simulink subsystem "EM"  (R2024a)
settings: Solver=VariableStepAuto  StartTime=0.0  StopTime=10.0  RelTol=1e-3
settings Model: Creator=Dell  LastModifiedBy=mrvol

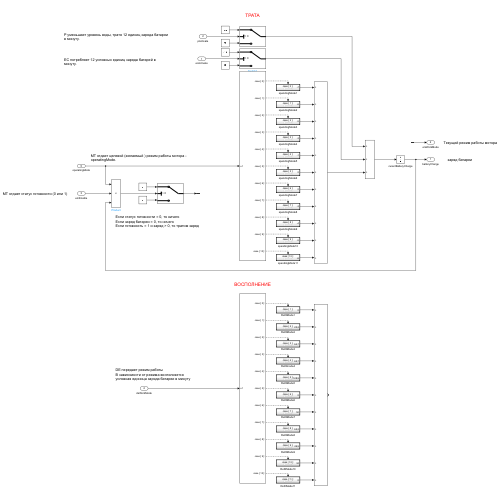
[thumbnail: Simulink's stored preview of the top-level diagram]
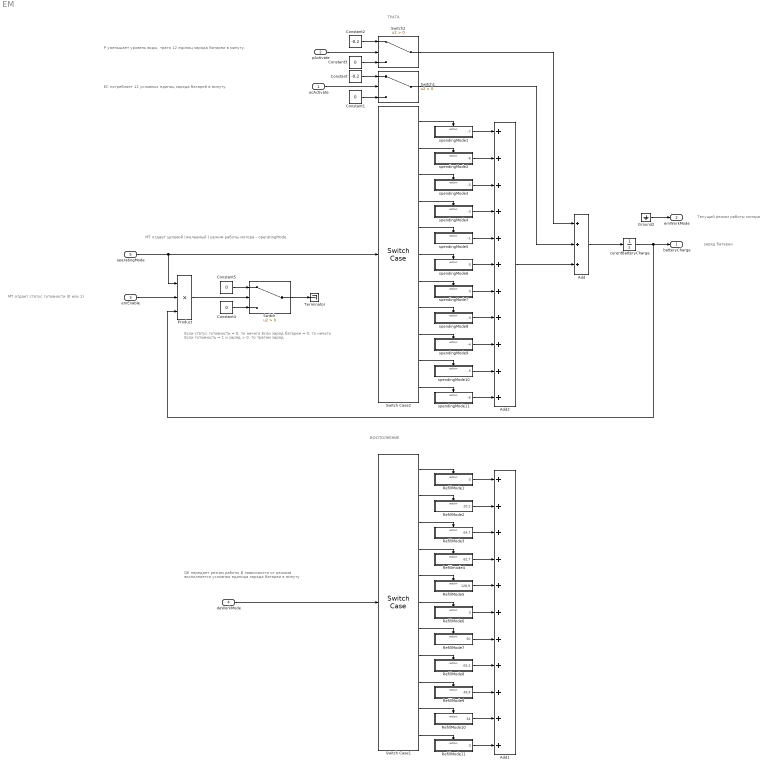
== system EM ==
  note: Если статус готовности = 0, то ничего
      | Если заряд батареи = 0, то ничего
      | Если готовность = 1 и заряд > 0, то тратим заряд
  note: ВОСПОЛНЕНИЕ
  note: ТРАТА
  note: EC потребляет 12 условных единиц заряда батарей в минуту.
  note: Текущий режим работы мотора
  note: заряд батареи
  note: P уменьшает уровень воды, тратя 12 единиц заряда батареи в минуту.
  note: MT отдает статус готовности (0 или 1)
  note: MT отдает целевой (желаемый ) режим работы мотора - operatingMode.
  note: DE передает режим работы
      | В зависомости от режима восполняется
      | условная единица заряда батареи в минуту
  ecActivate : Inport
  pActivate : Inport  Port=2
  emEnable : Inport  Port=3
  deWorkMode : Inport  Port=4
  operatingMode : Inport  Port=5
  Add : Sum  Inputs=+++
  Add1 : Sum  Inputs=+++++++++++
  Add2 : Sum  Inputs=+++++++++++
  Constant : Constant  Value=-0.2
  Constant{1,3..5} (4 alike) : Constant  Value=0
  Constant2 : Constant  Value=-0.2
  Ground2 : Ground
  Product : Product  Inputs=3
  RefillMode1 : Subsystem  TreatAsAtomicUnit=on
  RefillMode10 : Subsystem  TreatAsAtomicUnit=on
  RefillMode11 : Subsystem  TreatAsAtomicUnit=on
  RefillMode2 : Subsystem  TreatAsAtomicUnit=on
  RefillMode3 : Subsystem  TreatAsAtomicUnit=on
  RefillMode5 : Subsystem  TreatAsAtomicUnit=on
  RefillMode6 : Subsystem  TreatAsAtomicUnit=on
  RefillMode7 : Subsystem  TreatAsAtomicUnit=on
  RefillMode8 : Subsystem  TreatAsAtomicUnit=on
  RefillMode9 : Subsystem  TreatAsAtomicUnit=on
  Refillmode4 : Subsystem  TreatAsAtomicUnit=on
  Switch : Switch  Criteria=u2 > Threshold  SaturateOnIntegerOverflow=off  InputSameDT=off
  Switch Case1 : SwitchCase  CaseConditions={0, 1, 2, 3, 4, 5, 6, 7, 8, 9, 10}  ShowDefaultCase=off
  Switch Case2 : SwitchCase  CaseConditions={0, 1, 2, 3, 4, 5, 6, 7, 8, 9, 10}  ShowDefaultCase=off
  Switch1 : Switch  Criteria=u2 > Threshold  SaturateOnIntegerOverflow=off  InputSameDT=off
  Switch2 : Switch  Criteria=u2 > Threshold  SaturateOnIntegerOverflow=off  InputSameDT=off
  Terminator : Terminator
  curentBatteryCharge : Integrator
  spendingMode1 : Subsystem  TreatAsAtomicUnit=on
  spendingMode10 : Subsystem  TreatAsAtomicUnit=on
  spendingMode11 : Subsystem  TreatAsAtomicUnit=on
  spendingMode2 : Subsystem  TreatAsAtomicUnit=on
  spendingMode3 : Subsystem  TreatAsAtomicUnit=on
  spendingMode4 : Subsystem  TreatAsAtomicUnit=on
  spendingMode5 : Subsystem  TreatAsAtomicUnit=on
  spendingMode6 : Subsystem  TreatAsAtomicUnit=on
  spendingMode7 : Subsystem  TreatAsAtomicUnit=on
  spendingMode8 : Subsystem  TreatAsAtomicUnit=on
  spendingMode9 : Subsystem  TreatAsAtomicUnit=on
  batteryCharge : Outport
  emWorkMode : Outport  Port=2
  wires:
  Ground2/1 -> emWorkMode/1
  ecActivate/1 -> Switch1/2
  Constant/1 -> Switch1/1
  Constant1/1 -> Switch1/3
  pActivate/1 -> Switch2/2
  Constant2/1 -> Switch2/1
  Constant3/1 -> Switch2/3
  Constant4/1 -> Switch/3
  Constant5/1 -> Switch/1
  Refillmode4/1(62,7) -> Add1/4
  RefillMode8/1(65,2) -> Add1/8
  RefillMode5/1(128,9) -> Add1/5
  RefillMode2/1(20,2) -> Add1/2
  RefillMode3/1(64,7) -> Add1/3
  RefillMode6/1(0) -> Add1/6
  RefillMode10/1(34) -> Add1/10
  RefillMode9/1(49,9) -> Add1/9
  RefillMode1/1(0) -> Add1/1
  RefillMode7/1(50) -> Add1/7
  Switch Case1/7 -> RefillMode7/Action
  Switch Case1/5 -> RefillMode5/Action
  RefillMode11/1(0) -> Add1/11
  Switch Case1/3 -> RefillMode3/Action
  Switch Case1/11 -> RefillMode11/Action
  Switch Case1/8 -> RefillMode8/Action
  Switch Case1/6 -> RefillMode6/Action
  Switch Case1/4 -> Refillmode4/Action
  Switch Case1/1 -> RefillMode1/Action
  Switch Case1/10 -> RefillMode10/Action
  Switch Case1/9 -> RefillMode9/Action
  Switch Case1/2 -> RefillMode2/Action
  deWorkMode/1 -> Switch Case1/1
  Product/1 -> Switch/2
  Switch2/1 -> Add/1
  Switch1/1 -> Add/2
  Add/1 -> curentBatteryCharge/1
  Switch Case2/1 -> spendingMode1/Action
  Switch Case2/10 -> spendingMode10/Action
  Switch Case2/9 -> spendingMode9/Action
  spendingMode7/1(0) -> Add2/7
  Switch Case2/8 -> spendingMode8/Action
  Switch Case2/7 -> spendingMode7/Action
  Switch Case2/6 -> spendingMode6/Action
  Switch Case2/5 -> spendingMode5/Action
  Switch Case2/11 -> spendingMode11/Action
  Switch Case2/3 -> spendingMode3/Action
  Switch Case2/4 -> spendingMode4/Action
  spendingMode11/1(-6) -> Add2/11
  spendingMode9/1(-4) -> Add2/9
  spendingMode2/1(-6) -> Add2/2
  spendingMode1/1(-7) -> Add2/1
  spendingMode10/1(-5) -> Add2/10
  spendingMode6/1(0) -> Add2/6
  spendingMode3/1(-5) -> Add2/3
  spendingMode8/1(-3) -> Add2/8
  spendingMode4/1(-3) -> Add2/4
  Switch Case2/2 -> spendingMode2/Action
  spendingMode5/1(-1) -> Add2/5
  Add2/1 -> Add/3
  curentBatteryCharge/1 -> Product/3, batteryCharge/1
  operatingMode/1 -> Switch Case2/1, Product/1
  emEnable/1 -> Product/2
  Switch/1 -> Terminator/1

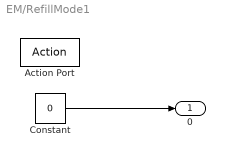
== system EM/RefillMode1 ==
  Action Port : ActionPort  ActionPortLabel=case [ 1 ]:
  Constant : Constant  Value=0
  0 : Outport
  wires:
  Constant/1 -> 0/1

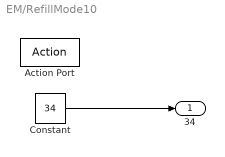
== system EM/RefillMode10 ==
  Action Port : ActionPort  ActionPortLabel=case [ 10 ]:
  Constant : Constant  Value=34
  34 : Outport
  wires:
  Constant/1 -> 34/1

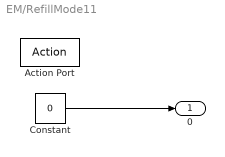
== system EM/RefillMode11 ==
  Action Port : ActionPort  ActionPortLabel=case [ 11 ]:
  Constant : Constant  Value=0
  0 : Outport
  wires:
  Constant/1 -> 0/1

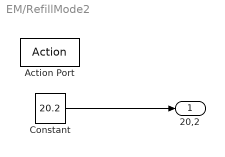
== system EM/RefillMode2 ==
  Action Port : ActionPort  ActionPortLabel=case [ 2 ]:
  Constant : Constant  Value=20.2
  20,2 : Outport
  wires:
  Constant/1 -> 20,2/1

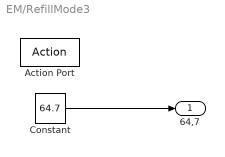
== system EM/RefillMode3 ==
  Action Port : ActionPort  ActionPortLabel=case [ 3 ]:
  Constant : Constant  Value=64.7
  64,7 : Outport
  wires:
  Constant/1 -> 64,7/1

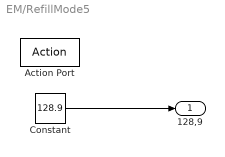
== system EM/RefillMode5 ==
  Action Port : ActionPort  ActionPortLabel=case [ 5 ]:
  Constant : Constant  Value=128.9
  128,9 : Outport
  wires:
  Constant/1 -> 128,9/1

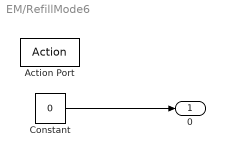
== system EM/RefillMode6 ==
  Action Port : ActionPort  ActionPortLabel=case [ 6 ]:
  Constant : Constant  Value=0
  0 : Outport
  wires:
  Constant/1 -> 0/1

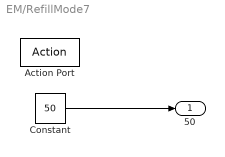
== system EM/RefillMode7 ==
  Action Port : ActionPort  ActionPortLabel=case [ 7 ]:
  Constant : Constant  Value=50
  50 : Outport
  wires:
  Constant/1 -> 50/1

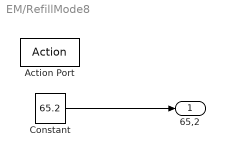
== system EM/RefillMode8 ==
  Action Port : ActionPort  ActionPortLabel=case [ 8 ]:
  Constant : Constant  Value=65.2
  65,2 : Outport
  wires:
  Constant/1 -> 65,2/1

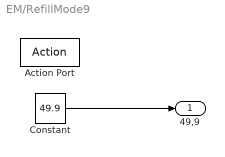
== system EM/RefillMode9 ==
  Action Port : ActionPort  ActionPortLabel=case [ 9 ]:
  Constant : Constant  Value=49.9
  49,9 : Outport
  wires:
  Constant/1 -> 49,9/1

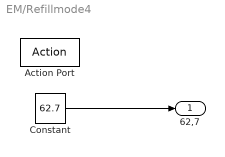
== system EM/Refillmode4 ==
  Action Port : ActionPort  ActionPortLabel=case [ 4 ]:
  Constant : Constant  Value=62.7
  62,7 : Outport
  wires:
  Constant/1 -> 62,7/1

== system EM/spendingMode1 ==
  Action Port : ActionPort  ActionPortLabel=case [ 0 ]:
  Constant : Constant  Value=-7
  -7 : Outport
  wires:
  Constant/1 -> -7/1

== system EM/spendingMode10 ==
  Action Port : ActionPort  ActionPortLabel=case [ 9 ]:
  Constant : Constant  Value=-5
  -5 : Outport
  wires:
  Constant/1 -> -5/1

== system EM/spendingMode11 ==
  Action Port : ActionPort  ActionPortLabel=case [ 10 ]:
  Constant : Constant  Value=-6
  -6 : Outport
  wires:
  Constant/1 -> -6/1

== system EM/spendingMode2 ==
  Action Port : ActionPort  ActionPortLabel=case [ 1 ]:
  Constant : Constant  Value=-6
  -6 : Outport
  wires:
  Constant/1 -> -6/1

== system EM/spendingMode3 ==
  Action Port : ActionPort  ActionPortLabel=case [ 2 ]:
  Constant : Constant  Value=-5
  -5 : Outport
  wires:
  Constant/1 -> -5/1

== system EM/spendingMode4 ==
  Action Port : ActionPort  ActionPortLabel=case [ 3 ]:
  Constant : Constant  Value=-3
  -3 : Outport
  wires:
  Constant/1 -> -3/1

== system EM/spendingMode5 ==
  Action Port : ActionPort  ActionPortLabel=case [ 4 ]:
  Constant : Constant  Value=-1
  -1 : Outport
  wires:
  Constant/1 -> -1/1

== system EM/spendingMode6 ==
  Action Port : ActionPort  ActionPortLabel=case [ 5 ]:
  Constant : Constant  Value=0
  0 : Outport
  wires:
  Constant/1 -> 0/1

== system EM/spendingMode7 ==
  Action Port : ActionPort  ActionPortLabel=case [ 6 ]:
  Constant : Constant  Value=0
  0 : Outport
  wires:
  Constant/1 -> 0/1

== system EM/spendingMode8 ==
  Action Port : ActionPort  ActionPortLabel=case [ 7 ]:
  Constant : Constant  Value=-3
  -3 : Outport
  wires:
  Constant/1 -> -3/1

== system EM/spendingMode9 ==
  Action Port : ActionPort  ActionPortLabel=case [ 8 ]:
  Constant : Constant  Value=-4
  -4 : Outport
  wires:
  Constant/1 -> -4/1
